simulink model "my_brake_throttle_sensor"  (R2024a)
settings: Solver=FixedStepDiscrete  StartTime=0.0  StopTime=10.0  FixedStep=0.005  RelTol=1e-3
model workspace (MATLAB code in the model file):
  | TPSPercent_LkupTbl = Simulink.LookupTable;
  | TPSPercent_LkupTbl.Table.DataType = 'single';
  | TPSPercent_LkupTbl.Table.Min = [];
  | TPSPercent_LkupTbl.Table.Max = [];
  | TPSPercent_LkupTbl.Table.Unit = '';
  | TPSPercent_LkupTbl.Table.FieldName = 'Table';
  | TPSPercent_LkupTbl.Table.Description = '';
  | TPSPercent_LkupTbl.Table.Value = ...
  |   [0 10 20 30 40 50 60 70 80 90 100];
  | TPSPercent_LkupTbl.BreakpointsSpecification = 'Explicit values';
  | TPSPercent_LkupTbl.SupportTunableSize = false;
  | TPSPercent_LkupTbl.Breakpoints.DataType = 'single';
  | TPSPercent_LkupTbl.Breakpoints.Min = [];
  | TPSPercent_LkupTbl.Breakpoints.Max = [];
  | TPSPercent_LkupTbl.Breakpoints.Unit = '';
  | TPSPercent_LkupTbl.Breakpoints.FieldName = 'BP1';
  | TPSPercent_LkupTbl.Breakpoints.Description = '';
  | TPSPercent_LkupTbl.Breakpoints.Value = single(linspace(170, 966, 11));
  | TPSPercent_LkupTbl.Breakpoints.TunableSizeName = 'N1';
  | TPSPercent_LkupTbl.CoderInfo.StorageClass = 'Auto';
  | TPSPercent_LkupTbl.StructTypeInfo.Name = 'MyStruct';
  | TPSPercent_LkupTbl.StructTypeInfo.DataScope = 'Auto';
  | TPSPercent_LkupTbl.StructTypeInfo.HeaderFileName = 'Rte_Type.h';
undefined symbols (not defined in the file or in its folder): TPSPercentBkpt, TPSPercentTbl
settings Model: ParameterArgumentNames=TPSPercent_LkupTbl  Creator=The MathWorks, Inc.  LastModifiedBy=Mhamed
settings SolverCC: AlgebraicLoopSolver=TrustRegion  MaxZcPerStep=1
settings DataIOCC: SaveFormat=StructureWithTime  ReturnWorkspaceOutputs=off
settings OptimizationCC: DefaultParameterBehavior=Inlined  ReuseModelBlockBuffer=off  PassReuseOutputArgsAs=Individual arguments  ZeroExternalMemoryAtStartup=off  ZeroInternalMemoryAtStartup=off  EfficientTunableParamExpr=on
settings DebuggingCC: ParameterTunabilityLossMsg=error  UnconnectedInputMsg=warning  UnconnectedOutputMsg=warning  UnconnectedLineMsg=warning  ArithmeticOperatorsInVariantConditions=warning
settings ModelReferenceCC: EnableRefExpFcnMdlSchedulingChecks=on
settings SFSimCC: SimUseLocalCustomCode=off  MATLABDynamicMemAlloc=off  CustomCodeUndefinedFunction=UseInterfaceOnly
settings RTWCC: Description=AUTOSAR  SystemTargetFile=autosar.tlc  GenCodeOnly=on  TemplateMakefile=ert_default_tmf  GenerateReport=on  RTWUseLocalCustomCode=off  IncludeHyperlinkInReport=on  LaunchReport=on  DataTypeReplacement=CDataTypesFixedWidth  GenerateTraceInfo=on  GenerateTraceReport=on  GenerateTraceReportSl=on  GenerateTraceReportSf=on  GenerateTraceReportEml=on  GPUComputeCapability=3.5
settings CodeAppCC: ForceParamTrailComments=on  IgnoreCustomStorageClasses=off  OperatorAnnotations=on  SimulinkDataObjDesc=on  SFDataObjDesc=on  InsertBlockDesc=on
settings STFCustomTargetCC: MultiwordLength=256  ParMdlRefBuildCompliant=on  CompOptLevelCompliant=on  IncludeMdlTerminateFcn=off  CombineOutputUpdateFcns=on  SuppressErrorStatus=on  ERTCustomFileBanners=on  CodeInterfacePackaging=Reusable function  SupportNonFinite=off  SupportComplex=off  SupportContinuousTime=off  SupportNonInlinedSFcns=off  RemoveResetFunc=on  MATLABClassNameForMDSCustomization=Simulink.SoftwareTarget.ERTCustomization  CPPClassGenCompliant=on  AutosarCompliant=on  GRTInterface=off  LookupTableObjectStructAxisOrder=2,1,3,4,...  LUTObjectStructOrderEvenSpacing=Size,Table,Breakpoints  SystemTargetFile=autosar.tlc
settings ERTTargetCC: TargetLangStandard=C99 (ISO)  ConcurrentExecutionCompliant=off  IncludeMdlTerminateFcn=off  SuppressErrorStatus=on  CodeInterfacePackaging=Reusable function  SupportNonFinite=off  SupportComplex=off  ModelStepFunctionPrototypeControlCompliant=off  AutosarCompliant=on  LookupTableObjectStructAxisOrder=2,1,3,4,...  LUTObjectStructOrderEvenSpacing=Size,Table,Breakpoints  InlinedParameterPlacement=NonHierarchical  ERTCustomFileTemplate=example_file_process.tlc  BooleanTrueId=TRUE  BooleanFalseId=FALSE

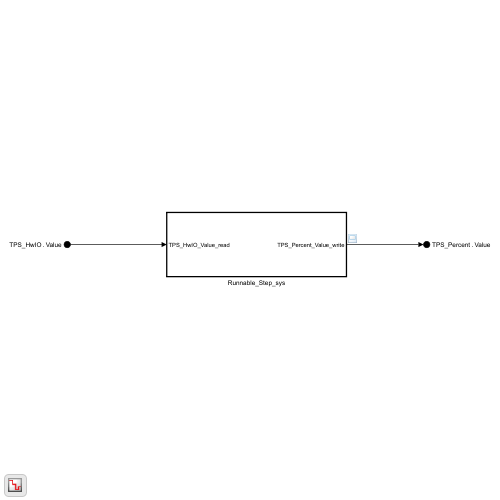
[thumbnail: Simulink's stored preview of the top-level diagram]
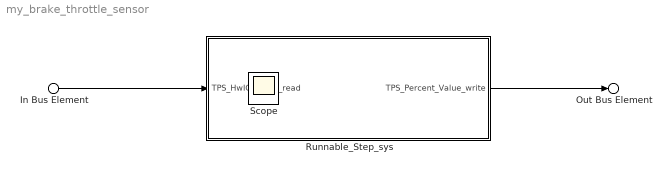
== system my_brake_throttle_sensor ==
  In Bus Element : Inport  PortName=TPS_HwIO  Element=Elem0
  Runnable_Step_sys : Subsystem  TreatAsAtomicUnit=on  SystemSampleTime=0.005
  Out Bus Element : Outport  PortName=TPS_Percent  Element=Value
  Scope : Scope
  wires:
  In Bus Element/1 -> Runnable_Step_sys/1(TPS_HwIO_Value_read)
  Runnable_Step_sys/1(TPS_Percent_Value_write) -> Out Bus Element/1

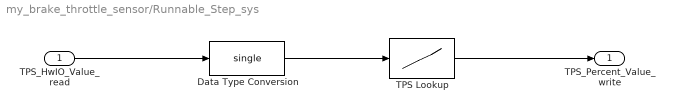
== system my_brake_throttle_sensor/Runnable_Step_sys ==
  TPS_HwIO_Value_read : Inport
  Data Type Conversion : DataTypeConversion  OutDataTypeStr=single  SaturateOnIntegerOverflow=off  RndMeth=Floor
  TPS Lookup : Lookup_n-D  NumberOfTableDimensions=1  DataSpecification=Lookup table object  LookupTableObject=TPSPercent_LkupTbl  BreakpointsForDimension1=TPSPercentBkpt  BreakpointsForDimension1DataTypeStr=single  IndexSearchMethod=Linear search  Table=TPSPercentTbl  TableDataTypeStr=single  ExtrapMethod=Clip  InternalRulePriority=Speed  OutDataTypeStr=single  RndMeth=Simplest
  TPS_Percent_Value_write : Outport  VectorParamsAs1DForOutWhenUnconnected=off
  wires:
  TPS_HwIO_Value_read/1 -> Data Type Conversion/1
  TPS Lookup/1 -> TPS_Percent_Value_write/1
  Data Type Conversion/1 -> TPS Lookup/1
